simulink model "controller"  (R2021b)
settings: Solver=FixedStepDiscrete  StartTime=0.0  StopTime=inf  FixedStep=1  RelTol=1e-3
model workspace (MAT data in the model file):
  callButtonPressedC1 = Simulink.Parameter
  callButtonPressedC1.Value = 0
  callButtonPressedC1.DataType = 'auto'
  callButtonPressedC1.Complexity = 'real'
  callButtonPressedC1.Dimensions = [1 1]
  callButtonPressedC2 = Simulink.Parameter
  callButtonPressedC2.Value = 0
  callButtonPressedC2.DataType = 'auto'
  callButtonPressedC2.Complexity = 'real'
  callButtonPressedC2.Dimensions = [1 1]
settings Model: Creator=chioma  LastModifiedBy=chioma
settings OptimizationCC: BlockReduction=off  DefaultParameterBehavior=Inlined  BufferReuse=off
settings ConfigComp: CovEnable=on  RecordCoverage=on  CovModelRefEnable=on

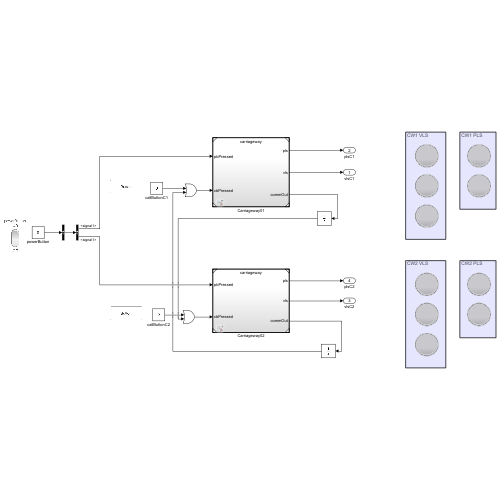
[thumbnail: Simulink's stored preview of the top-level diagram]
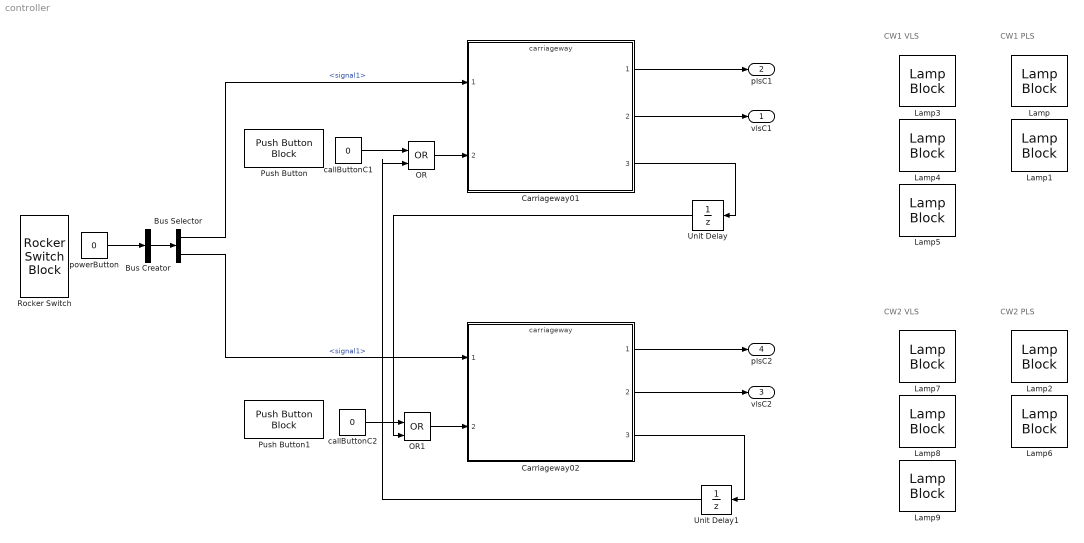
== system controller ==
  note: CW1 VLS
  note: CW1 PLS
  note: CW2 VLS
  note: CW2 PLS
  Bus Creator : BusCreator  Inputs=1
  Bus Selector : BusSelector  OutputSignals=signal1,signal1
  Carriageway01 : ModelReference  ModelNameDialog=carriageway.slx  SimulationMode=Normal  ModelReferenceVersion=1.24
  Carriageway02 : ModelReference  ModelNameDialog=carriageway.slx  SimulationMode=Normal  ModelReferenceVersion=1.24
  Lamp{,1..9} (10 alike) : LampBlock  LabelPosition=Hide
  OR : Logic  Operator=OR  IconShape=distinctive  AllPortsSameDT=off  OutDataTypeStr=boolean
  OR1 : Logic  Operator=OR  IconShape=distinctive  AllPortsSameDT=off  OutDataTypeStr=boolean
  Push Button : PushButtonBlock  OffValue=0.000000
  Push Button1 : PushButtonBlock  OffValue=0.000000
  Rocker Switch : RockerSwitchBlock
      settings: Values={{'Off', 'On'}, [0 1]}
  Unit Delay : UnitDelay  HasFrameUpgradeWarning=on
  Unit Delay1 : UnitDelay  HasFrameUpgradeWarning=on
  callButtonC1 : Constant  Value=0
  callButtonC2 : Constant  Value=0
  powerButton : Constant  Value=0  OutDataTypeStr=Inherit: Inherit via back propagation
  vlsC1 : Outport
  plsC1 : Outport  Port=2
  vlsC2 : Outport  Port=3
  plsC2 : Outport  Port=4
  wires:
  powerButton/1 -> Bus Creator/1
  Bus Selector/1 -> Carriageway01/1  "<signal1>"
  callButtonC2/1 -> OR1/1
  Bus Creator/1 -> Bus Selector/1
  Bus Selector/2 -> Carriageway02/1  "<signal1>"
  callButtonC1/1 -> OR/1
  Carriageway02/3 -> Unit Delay1/1
  Carriageway01/3 -> Unit Delay/1
  Unit Delay/1 -> OR1/2
  Unit Delay1/1 -> OR/2
  Carriageway01/1 -> plsC1/1
  Carriageway01/2 -> vlsC1/1
  Carriageway02/1 -> plsC2/1
  Carriageway02/2 -> vlsC2/1
  OR/1 -> Carriageway01/2
  OR1/1 -> Carriageway02/2
